simulink model "PMSM_drive_Simulink"  (R2024a)
settings: Solver=ode45  StartTime=0.0  StopTime=10.0  RelTol=1e-6  AbsTol=1e-8
values from neighbouring files (symbols this model uses):
  B = 0.08    [PMSM_drive_main_code.m]
  Ba = alfaw*J - B    (= 0.17)    [PMSM_drive_main_code.m]
  Beta0 = Beta_fixed*pi/180    (= 1.9753514301)    [PMSM_drive_main_code.m]
  Beta_step = 130*pi/180    (= 2.26892802759)    [PMSM_drive_main_code.m]
  Beta_time = 2.3    [PMSM_drive_main_code.m]
  Irated = 6.5*sqrt(2)    [PMSM_drive_main_code.m]
  isd0 = 0    [PMSM_drive_main_code.m]
  isq0 = 0    [PMSM_drive_main_code.m]
  J = 0.0125    [PMSM_drive_main_code.m]
  Kicd = alfac*(Rs+Rad)    (= 34500)    [PMSM_drive_main_code.m]
  Kicq = alfac*(Rs+Raq)    (= 85500)    [PMSM_drive_main_code.m]
  Kiw = alfaw*(B+Ba)    (= 5)    [PMSM_drive_main_code.m]
  Kpcd = alfac*Lsdhat    (= 34.5)    [PMSM_drive_main_code.m]
  Kpcq = alfac*Lsqhat    (= 85.5)    [PMSM_drive_main_code.m]
  Kpw = alfaw*J    (= 0.25)    [PMSM_drive_main_code.m]
  Lsd = Laa0+Lab0+3/2*Laa2    (= 0.0345)    [PMSM_drive_main_code.m]
  Lsq = Laa0+Lab0-3/2*Laa2    (= 0.0855)    [PMSM_drive_main_code.m]
  np = 2    [PMSM_drive_main_code.m]
  Psim = 0.822    [PMSM_drive_main_code.m]
  Rad = alfac*Lsdhat-Rs    (= 33.17)    [PMSM_drive_main_code.m]
  Raq = alfac*Lsqhat-Rs    (= 84.17)    [PMSM_drive_main_code.m]
  Rs = 1.33    [PMSM_drive_main_code.m]
  Te_ref = 16.6    [PMSM_drive_main_code.m]
  Te_ref2 = 4    [PMSM_drive_main_code.m]
  Te_ref_time = 0.1    [PMSM_drive_main_code.m]
  Te_ref_time2 = 2.7    [PMSM_drive_main_code.m]
  theta0 = 0    [PMSM_drive_main_code.m]
  TL_extra = 4    [PMSM_drive_main_code.m]
  TL_extra_time = 1.1    [PMSM_drive_main_code.m]
  Umax = 440*sqrt(2/3)    [PMSM_drive_main_code.m]
  usd0 = Rs*isd0-ws*Lsq*isq0    [PMSM_drive_main_code.m]
  usq0 = Rs*isq0+ws*Lsd*isd0+ws*Psim    [PMSM_drive_main_code.m]
  VconvLim = Umax    [PMSM_drive_main_code.m]
  wr0 = 0    [PMSM_drive_main_code.m]
  ws = 2*pi*fs    (= 314.159265359)    [PMSM_drive_main_code.m]
undefined symbols (not defined in the file or in its folder): j
settings Model: Creator=e6zebra  LastModifiedBy=munav
settings SolverCC: AutoScaleAbsTol=off  AlgebraicLoopSolver=TrustRegion
settings DataIOCC: SaveFormat=Array  SignalLoggingSaveFormat=ModelDataLogs  ReturnWorkspaceOutputs=off
settings OptimizationCC: BlockReduction=off  BooleanDataType=off  ExpressionDepthLimit=2147483647  InitFltsAndDblsToZero=on  LifeSpan=inf
settings DebuggingCC: SaveWithParameterizedLinksMsg=none  UnderspecifiedInitializationDetection=Classic  MergeDetectMultiDrivingBlocksExec=none  SignalResolutionControl=TryResolveAllWithWarning  MultiTaskDSMMsg=warning  MultiTaskCondExecSysMsg=none  FcnCallInpInsideContextMsg=warning  UnconnectedInputMsg=warning  UnconnectedOutputMsg=warning  UnconnectedLineMsg=warning  StateNameClashWarn=warning  SFUnexpectedBacktrackingDiag=warning  SFNoUnconditionalDefaultTransitionDiag=warning  SFExecutionAtInitializationDiag=none  ArithmeticOperatorsInVariantConditions=warning
settings HardwareCC: ProdBitPerPointer=32  ProdBitPerSizeT=32  ProdBitPerPtrDiffT=32  ProdLargestAtomicFloat=None  ProdIntDivRoundTo=Undefined  ProdEndianess=Unspecified  ProdWordSize=32  ProdHWDeviceType=32-bit Generic  TargetUnknown=on
settings ModelReferenceCC: EnableRefExpFcnMdlSchedulingChecks=on  PropagateSignalLabelsOutOfModel=off
settings SFSimCC: SimUseLocalCustomCode=off  CustomCodeUndefinedFunction=UseInterfaceOnly
settings RTWCC: TemplateMakefile=grt.tmf  RTWUseLocalCustomCode=off  GPUComputeCapability=3.5
settings CodeAppCC: StateflowObjectComments=on
settings GRTTargetCC: TargetFcnLib=ansi_tfl_tmw.mat  TargetLangStandard=C89/C90 (ANSI)  CombineOutputUpdateFcns=off  GRTInterface=on
settings ConfigComp: CovMetricSettings=dw  CovSaveCumulativeToWorkspaceVar=on  CovSaveSingleToWorkspaceVar=on  CovExternalEMLEnable=off

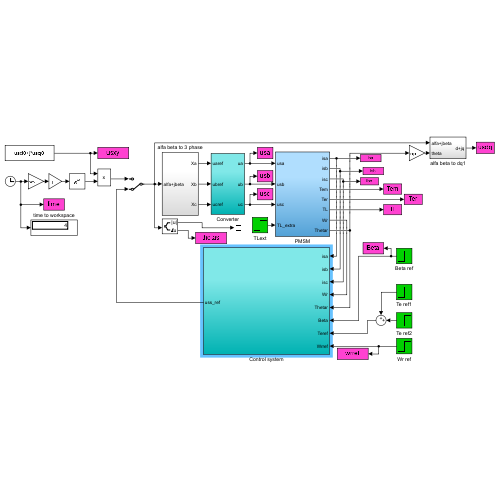
[thumbnail: Simulink's stored preview of the top-level diagram]
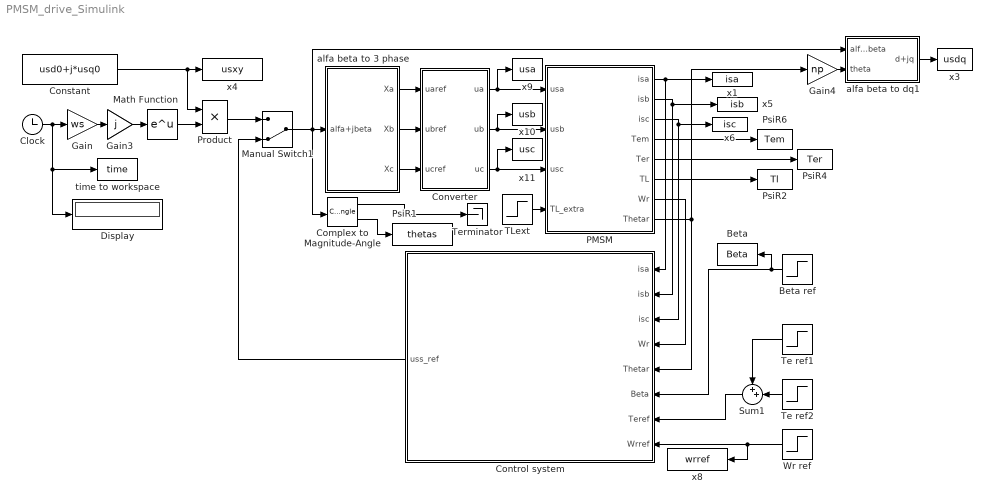
== system PMSM_drive_Simulink ==
  Beta : ToWorkspace  VariableName=Beta  SampleTime=-1
  Beta ref : Step  Time=Beta_time  Before=Beta0  After=Beta_step  SampleTime=0
  Clock : Clock
  Complex to Magnitude-Angle : ComplexToMagnitudeAngle
  Constant : Constant  Value=usd0+j*usq0
  Control system : Subsystem
  Converter : Subsystem
  Display : Display
  Gain : Gain  Gain=ws
  Gain3 : Gain  Gain=j  SaturateOnIntegerOverflow=on  OutDataTypeStr=Inherit: Same as input  ParamDataTypeStr=Inherit: Same as input
  Gain4 : Gain  Gain=np
  Manual Switch1 : ManualSwitch  CurrentSetting=0
  Math Function : Math  SignedPower=on
  PMSM : Subsystem
  Product : Product  SaturateOnIntegerOverflow=on  OutDataTypeStr=Inherit: Same as first input
  PsiR1 : ToWorkspace  VariableName=thetas  SampleTime=-1
  PsiR2 : ToWorkspace  VariableName=Tl  SampleTime=-1
  PsiR4 : ToWorkspace  VariableName=Ter  SampleTime=-1
  PsiR6 : ToWorkspace  VariableName=Tem  SampleTime=-1
  Sum1 : Sum  Inputs=++|  SaturateOnIntegerOverflow=on
  TLext : Step  Time=TL_extra_time  After=TL_extra  SampleTime=0
  Te ref1 : Step  Time=Te_ref_time  After=Te_ref  SampleTime=0
  Te ref2 : Step  Time=Te_ref_time2  After=Te_ref2  SampleTime=0
  Terminator : Terminator
  Wr ref : Step  After=1435*pi/30  SampleTime=0
  alfa beta to 3 phase : Subsystem
  alfa beta to dq1 : Subsystem
  time to workspace : ToWorkspace  VariableName=time  SampleTime=-1
  x1 : ToWorkspace  VariableName=isa  SampleTime=-1
  x10 : ToWorkspace  VariableName=usb  SampleTime=-1
  x11 : ToWorkspace  VariableName=usc  SampleTime=-1
  x3 : ToWorkspace  VariableName=usdq  SampleTime=-1
  x4 : ToWorkspace  VariableName=usxy  SampleTime=-1
  x5 : ToWorkspace  VariableName=isb  SampleTime=-1
  x6 : ToWorkspace  VariableName=isc  SampleTime=-1
  x8 : ToWorkspace  VariableName=wrref  SampleTime=-1
  x9 : ToWorkspace  VariableName=usa  SampleTime=-1
  wires:
  Clock/1 -> Gain/1, time to workspace/1, Display/1
  TLext/1 -> PMSM/4(TL_extra)
  Beta ref/1 -> Control system/6(Beta), Beta/1
  Wr ref/1 -> x8/1, Control system/8(Wrref)
  Gain/1 -> Gain3/1
  Constant/1 -> x4/1, Product/1
  PMSM/8(Thetar) -> Control system/5(Thetar), Gain4/1
  PMSM/6(TL) -> PsiR2/1
  PMSM/5(Ter) -> PsiR4/1
  alfa beta to dq1/1(d+jq) -> x3/1
  Converter/1(ua) -> PMSM/1(usa), x9/1
  Converter/2(ub) -> PMSM/2(usb), x10/1
  Converter/3(uc) -> PMSM/3(usc), x11/1
  alfa beta to 3 phase/1(Xa) -> Converter/1(uaref)
  alfa beta to 3 phase/2(Xb) -> Converter/2(ubref)
  alfa beta to 3 phase/3(Xc) -> Converter/3(ucref)
  Gain3/1 -> Math Function/1
  Math Function/1 -> Product/2
  Complex to Magnitude-Angle/2 -> PsiR1/1
  Complex to Magnitude-Angle/1 -> Terminator/1
  Te ref1/1 -> Sum1/1
  Te ref2/1 -> Sum1/2
  Manual Switch1/1 -> alfa beta to 3 phase/1(alfa+jbeta), alfa beta to dq1/1(alfa+jbeta), Complex to Magnitude-Angle/1
  PMSM/4(Tem) -> PsiR6/1
  Product/1 -> Manual Switch1/1
  Gain4/1 -> alfa beta to dq1/2(theta)
  PMSM/2(isb) -> Control system/2(isb), x5/1
  PMSM/3(isc) -> Control system/3(isc), x6/1
  PMSM/7(Wr) -> Control system/4(Wr)
  Sum1/1 -> Control system/7(Teref)
  Control system/1(uss_ref) -> Manual Switch1/2
  PMSM/1(isa) -> Control system/1(isa), x1/1

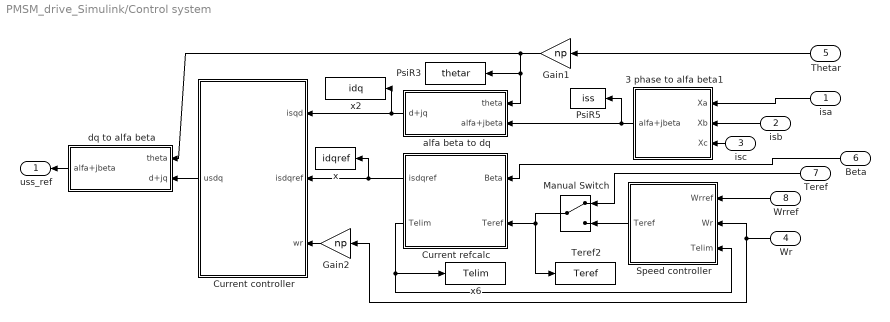
== system PMSM_drive_Simulink/Control system ==
  isa : Inport
  isb : Inport  Port=2
  isc : Inport  Port=3
  Wr : Inport  Port=4
  Thetar : Inport  Port=5
  Beta : Inport  Port=6
  Teref : Inport  Port=7
  Wrref : Inport  Port=8
  3 phase to alfa beta1 : Subsystem
  Current controller : Subsystem
  Current refcalc : Subsystem
  Gain1 : Gain  Gain=np
  Gain2 : Gain  Gain=np
  Manual Switch : ManualSwitch
  PsiR3 : ToWorkspace  VariableName=thetar  SampleTime=-1
  PsiR5 : ToWorkspace  VariableName=iss  SampleTime=-1
  Speed controller : Subsystem
  Teref2 : ToWorkspace  VariableName=Teref  SampleTime=-1
  alfa beta to dq : Subsystem
  dq to alfa beta : Subsystem
  x : ToWorkspace  VariableName=idqref  SampleTime=-1
  x2 : ToWorkspace  VariableName=idq  SampleTime=-1
  x6 : ToWorkspace  VariableName=Telim  SampleTime=-1
  uss_ref : Outport  VectorParamsAs1DForOutWhenUnconnected=off
  wires:
  Wr/1 -> Gain2/1, Speed controller/2(Wr)
  alfa beta to dq/1(d+jq) -> x2/1, Current controller/1(isqd)
  Current refcalc/1(isdqref) -> x/1, Current controller/2(isdqref)
  Current refcalc/2(Telim) -> Speed controller/3(Telim), x6/1
  Gain1/1 -> PsiR3/1, alfa beta to dq/1(theta), dq to alfa beta/1(theta)
  Gain2/1 -> Current controller/3(wr)
  isc/1 -> 3 phase to alfa beta1/3(Xc)
  isb/1 -> 3 phase to alfa beta1/2(Xb)
  isa/1 -> 3 phase to alfa beta1/1(Xa)
  3 phase to alfa beta1/1(alfa+jbeta) -> PsiR5/1, alfa beta to dq/2(alfa+jbeta)
  Current controller/1(usdq) -> dq to alfa beta/2(d+jq)
  Manual Switch/1 -> Current refcalc/2(Teref), Teref2/1
  dq to alfa beta/1(alfa+jbeta) -> uss_ref/1
  Thetar/1 -> Gain1/1
  Beta/1 -> Current refcalc/1(Beta)
  Wrref/1 -> Speed controller/1(Wrref)
  Teref/1 -> Manual Switch/1
  Speed controller/1(Teref) -> Manual Switch/2

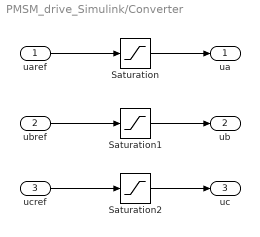
== system PMSM_drive_Simulink/Converter ==
  uaref : Inport
  ubref : Inport  Port=2
  ucref : Inport  Port=3
  Saturation : Saturate  UpperLimit=VconvLim  LowerLimit=-VconvLim
  Saturation1 : Saturate  UpperLimit=VconvLim  LowerLimit=-VconvLim
  Saturation2 : Saturate  UpperLimit=VconvLim  LowerLimit=-VconvLim
  ua : Outport  VectorParamsAs1DForOutWhenUnconnected=off
  ub : Outport  Port=2  VectorParamsAs1DForOutWhenUnconnected=off
  uc : Outport  Port=3  VectorParamsAs1DForOutWhenUnconnected=off
  wires:
  Saturation2/1 -> uc/1
  Saturation1/1 -> ub/1
  Saturation/1 -> ua/1
  uaref/1 -> Saturation/1
  ubref/1 -> Saturation1/1
  ucref/1 -> Saturation2/1

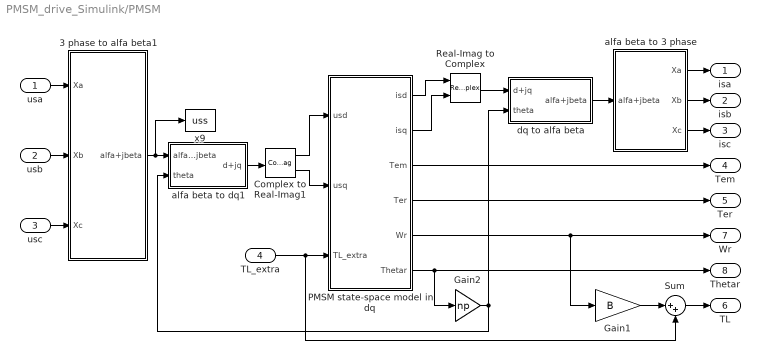
== system PMSM_drive_Simulink/PMSM ==
  usa : Inport
  usb : Inport  Port=2
  usc : Inport  Port=3
  TL_extra : Inport  Port=4
  3 phase to alfa beta1 : Subsystem
  Complex to Real-Imag1 : ComplexToRealImag
  Gain1 : Gain  Gain=B
  Gain2 : Gain  Gain=np
  PMSM state-space model in dq : Subsystem
  Real-Imag to Complex : RealImagToComplex
  Sum : Sum  Inputs=|++  SaturateOnIntegerOverflow=on
  alfa beta to 3 phase : Subsystem
  alfa beta to dq1 : Subsystem
  dq to alfa beta : Subsystem
  x9 : ToWorkspace  VariableName=uss  SampleTime=-1
  isa : Outport  VectorParamsAs1DForOutWhenUnconnected=off
  isb : Outport  Port=2  VectorParamsAs1DForOutWhenUnconnected=off
  isc : Outport  Port=3  VectorParamsAs1DForOutWhenUnconnected=off
  Tem : Outport  Port=4  VectorParamsAs1DForOutWhenUnconnected=off
  Ter : Outport  Port=5  VectorParamsAs1DForOutWhenUnconnected=off
  TL : Outport  Port=6  VectorParamsAs1DForOutWhenUnconnected=off
  Wr : Outport  Port=7  VectorParamsAs1DForOutWhenUnconnected=off
  Thetar : Outport  Port=8  VectorParamsAs1DForOutWhenUnconnected=off
  wires:
  TL_extra/1 -> Sum/2, PMSM state-space model in dq/3(TL_extra)
  Gain1/1 -> Sum/1
  Sum/1 -> TL/1
  usc/1 -> 3 phase to alfa beta1/3(Xc)
  usb/1 -> 3 phase to alfa beta1/2(Xb)
  usa/1 -> 3 phase to alfa beta1/1(Xa)
  alfa beta to 3 phase/1(Xa) -> isa/1
  alfa beta to 3 phase/3(Xc) -> isc/1
  alfa beta to 3 phase/2(Xb) -> isb/1
  Real-Imag to Complex/1 -> dq to alfa beta/1(d+jq)
  dq to alfa beta/1(alfa+jbeta) -> alfa beta to 3 phase/1(alfa+jbeta)
  alfa beta to dq1/1(d+jq) -> Complex to Real-Imag1/1
  PMSM state-space model in dq/5(Wr) -> Gain1/1, Wr/1
  PMSM state-space model in dq/6(Thetar) -> Gain2/1, Thetar/1
  Complex to Real-Imag1/1 -> PMSM state-space model in dq/1(usd)
  Complex to Real-Imag1/2 -> PMSM state-space model in dq/2(usq)
  PMSM state-space model in dq/1(isd) -> Real-Imag to Complex/1
  PMSM state-space model in dq/2(isq) -> Real-Imag to Complex/2
  PMSM state-space model in dq/3(Tem) -> Tem/1
  PMSM state-space model in dq/4(Ter) -> Ter/1
  Gain2/1 -> alfa beta to dq1/2(theta), dq to alfa beta/2(theta)
  3 phase to alfa beta1/1(alfa+jbeta) -> x9/1, alfa beta to dq1/1(alfa+jbeta)

== system PMSM_drive_Simulink/alfa beta to 3 phase ==
  alfa+jbeta : Inport
  Add1 : Sum  Inputs=-+
  Add2 : Sum  Inputs=--
  Complex to Real-Imag : ComplexToRealImag
  Gain1 : Gain  Gain=sqrt(3)/2
  Gain2 : Gain  Gain=1/2
  Xa : Outport  VectorParamsAs1DForOutWhenUnconnected=off
  Xb : Outport  Port=2  VectorParamsAs1DForOutWhenUnconnected=off
  Xc : Outport  Port=3  VectorParamsAs1DForOutWhenUnconnected=off
  wires:
  alfa+jbeta/1 -> Complex to Real-Imag/1
  Complex to Real-Imag/1 -> Xa/1, Gain2/1
  Add2/1 -> Xc/1
  Add1/1 -> Xb/1
  Complex to Real-Imag/2 -> Gain1/1
  Gain1/1 -> Add1/2, Add2/2
  Gain2/1 -> Add1/1, Add2/1

== system PMSM_drive_Simulink/alfa beta to dq1 ==
  alfa+jbeta : Inport
  theta : Inport  Port=2
  Gain : Gain  Gain=-j  SaturateOnIntegerOverflow=on  OutDataTypeStr=Inherit: Same as input  ParamDataTypeStr=Inherit: Same as input
  Math Function : Math  SignedPower=on
  Product : Product  SaturateOnIntegerOverflow=on  OutDataTypeStr=Inherit: Same as first input
  d+jq : Outport  VectorParamsAs1DForOutWhenUnconnected=off
  wires:
  theta/1 -> Gain/1
  Gain/1 -> Math Function/1
  Math Function/1 -> Product/2
  alfa+jbeta/1 -> Product/1
  Product/1 -> d+jq/1

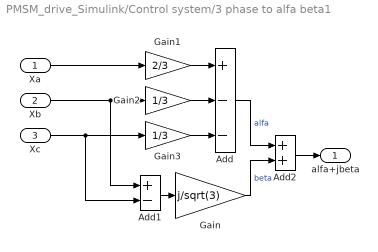
== system PMSM_drive_Simulink/Control system/3 phase to alfa beta1 ==
  Xa : Inport
  Xb : Inport  Port=2
  Xc : Inport  Port=3
  Add : Sum  Inputs=+--
  Add1 : Sum  Inputs=+-
  Add2 : Sum
  Gain : Gain  Gain=j/sqrt(3)
  Gain1 : Gain  Gain=2/3
  Gain2 : Gain  Gain=1/3
  Gain3 : Gain  Gain=1/3
  alfa+jbeta : Outport  VectorParamsAs1DForOutWhenUnconnected=off
  wires:
  Add1/1 -> Gain/1
  Add2/1 -> alfa+jbeta/1
  Gain/1 -> Add2/2  "beta"
  Add/1 -> Add2/1  "alfa"
  Gain3/1 -> Add/3
  Gain2/1 -> Add/2
  Gain1/1 -> Add/1
  Xa/1 -> Gain1/1
  Xb/1 -> Gain2/1, Add1/1
  Xc/1 -> Gain3/1, Add1/2

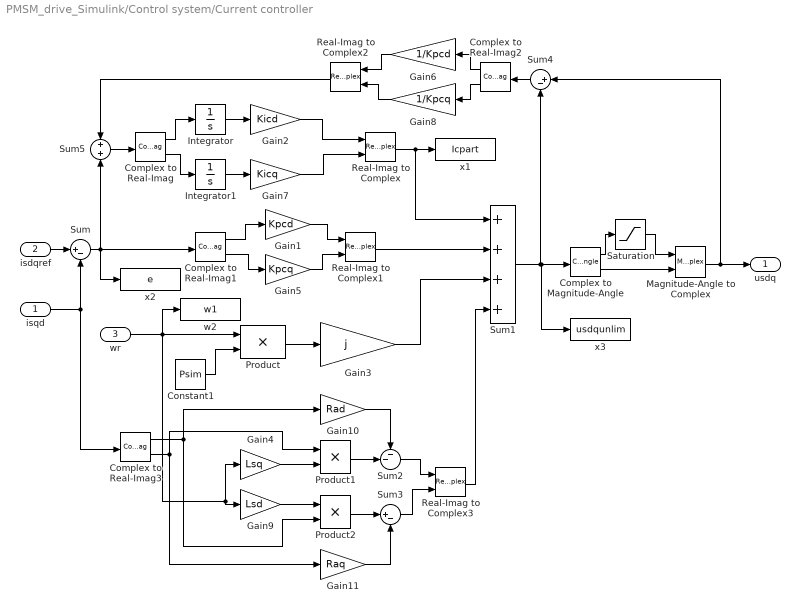
== system PMSM_drive_Simulink/Control system/Current controller ==
  isqd : Inport
  isdqref : Inport  Port=2
  wr : Inport  Port=3
  Complex to Magnitude-Angle : ComplexToMagnitudeAngle
  Complex to Real-Imag{,1..3} (4 alike) : ComplexToRealImag
  Constant1 : Constant  Value=Psim
  Gain1 : Gain  Gain=Kpcd  SaturateOnIntegerOverflow=on  OutDataTypeStr=Inherit: Same as input  ParamDataTypeStr=Inherit: Same as input
  Gain10 : Gain  Gain=Rad  SaturateOnIntegerOverflow=on  OutDataTypeStr=Inherit: Same as input  ParamDataTypeStr=Inherit: Same as input
  Gain11 : Gain  Gain=Raq  SaturateOnIntegerOverflow=on  OutDataTypeStr=Inherit: Same as input  ParamDataTypeStr=Inherit: Same as input
  Gain2 : Gain  Gain=Kicd  SaturateOnIntegerOverflow=on  OutDataTypeStr=Inherit: Same as input  ParamDataTypeStr=Inherit: Same as input
  Gain3 : Gain  Gain=j  SaturateOnIntegerOverflow=on  OutDataTypeStr=Inherit: Same as input  ParamDataTypeStr=Inherit: Same as input
  Gain4 : Gain  Gain=Lsq  SaturateOnIntegerOverflow=on  OutDataTypeStr=Inherit: Same as input  ParamDataTypeStr=Inherit: Same as input
  Gain5 : Gain  Gain=Kpcq  SaturateOnIntegerOverflow=on  OutDataTypeStr=Inherit: Same as input  ParamDataTypeStr=Inherit: Same as input
  Gain6 : Gain  Gain=1/Kpcd  SaturateOnIntegerOverflow=on  OutDataTypeStr=Inherit: Same as input  ParamDataTypeStr=Inherit: Same as input
  Gain7 : Gain  Gain=Kicq  SaturateOnIntegerOverflow=on  OutDataTypeStr=Inherit: Same as input  ParamDataTypeStr=Inherit: Same as input
  Gain8 : Gain  Gain=1/Kpcq  SaturateOnIntegerOverflow=on  OutDataTypeStr=Inherit: Same as input  ParamDataTypeStr=Inherit: Same as input
  Gain9 : Gain  Gain=Lsd  SaturateOnIntegerOverflow=on  OutDataTypeStr=Inherit: Same as input  ParamDataTypeStr=Inherit: Same as input
  Integrator : Integrator
  Integrator1 : Integrator
  Magnitude-Angle to Complex : MagnitudeAngleToComplex
  Product : Product  SaturateOnIntegerOverflow=on  OutDataTypeStr=Inherit: Same as first input
  Product1 : Product  SaturateOnIntegerOverflow=on  OutDataTypeStr=Inherit: Same as first input
  Product2 : Product  SaturateOnIntegerOverflow=on  OutDataTypeStr=Inherit: Same as first input
  Real-Imag to Complex{,1..3} (4 alike) : RealImagToComplex
  Saturation : Saturate  UpperLimit=Umax  LowerLimit=0
  Sum : Sum  Inputs=|+-  SaturateOnIntegerOverflow=on
  Sum1 : Sum  Inputs=++++  SaturateOnIntegerOverflow=on
  Sum2 : Sum  Inputs=--|  SaturateOnIntegerOverflow=on
  Sum3 : Sum  Inputs=|+-  SaturateOnIntegerOverflow=on
  Sum4 : Sum  Inputs=|+-  SaturateOnIntegerOverflow=on
  Sum5 : Sum  SaturateOnIntegerOverflow=on
  w2 : ToWorkspace  VariableName=w1  SampleTime=-1
  x1 : ToWorkspace  VariableName=Icpart  SampleTime=-1
  x2 : ToWorkspace  VariableName=e  SampleTime=-1
  x3 : ToWorkspace  VariableName=usdqunlim  SampleTime=-1
  usdq : Outport  VectorParamsAs1DForOutWhenUnconnected=off
  wires:
  isdqref/1 -> Sum/1
  isqd/1 -> Sum/2, Complex to Real-Imag3/1
  Sum/1 -> x2/1, Complex to Real-Imag1/1, Sum5/2
  Sum1/1 -> Complex to Magnitude-Angle/1, x3/1, Sum4/2
  Complex to Magnitude-Angle/1 -> Saturation/1
  Saturation/1 -> Magnitude-Angle to Complex/1
  Complex to Magnitude-Angle/2 -> Magnitude-Angle to Complex/2
  Magnitude-Angle to Complex/1 -> usdq/1, Sum4/1
  Complex to Real-Imag/2 -> Integrator1/1
  Complex to Real-Imag/1 -> Integrator/1
  Integrator/1 -> Gain2/1
  Integrator1/1 -> Gain7/1
  Real-Imag to Complex/1 -> Sum1/1, x1/1
  Product/1 -> Gain3/1
  Constant1/1 -> Product/2
  Gain4/1 -> Product1/2
  Gain3/1 -> Sum1/3
  Sum4/1 -> Complex to Real-Imag2/1
  Sum5/1 -> Complex to Real-Imag/1
  Real-Imag to Complex2/1 -> Sum5/1
  Complex to Real-Imag1/1 -> Gain1/1
  Real-Imag to Complex1/1 -> Sum1/2
  Gain1/1 -> Real-Imag to Complex1/1
  Complex to Real-Imag1/2 -> Gain5/1
  Gain5/1 -> Real-Imag to Complex1/2
  Gain2/1 -> Real-Imag to Complex/1
  Gain7/1 -> Real-Imag to Complex/2
  Complex to Real-Imag2/1 -> Gain6/1
  Gain6/1 -> Real-Imag to Complex2/1
  Complex to Real-Imag2/2 -> Gain8/1
  Gain8/1 -> Real-Imag to Complex2/2
  wr/1 -> w2/1, Gain4/1, Gain9/1, Product/1
  Real-Imag to Complex3/1 -> Sum1/4
  Complex to Real-Imag3/2 -> Product1/1, Gain11/1
  Sum2/1 -> Real-Imag to Complex3/1
  Gain9/1 -> Product2/1
  Complex to Real-Imag3/1 -> Product2/2, Gain10/1
  Product1/1 -> Sum2/2
  Gain10/1 -> Sum2/1
  Product2/1 -> Sum3/1
  Sum3/1 -> Real-Imag to Complex3/2
  Gain11/1 -> Sum3/2

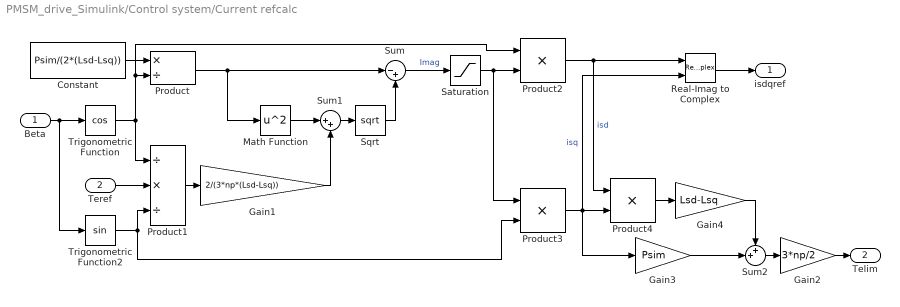
== system PMSM_drive_Simulink/Control system/Current refcalc ==
  Beta : Inport
  Teref : Inport  Port=2
  Constant : Constant  Value=Psim/(2*(Lsd-Lsq))
  Gain1 : Gain  Gain=2/(3*np*(Lsd-Lsq))  SaturateOnIntegerOverflow=on  OutDataTypeStr=Inherit: Same as input  ParamDataTypeStr=Inherit: Same as input
  Gain2 : Gain  Gain=3*np/2  SaturateOnIntegerOverflow=on  OutDataTypeStr=Inherit: Same as input  ParamDataTypeStr=Inherit: Same as input
  Gain3 : Gain  Gain=Psim  SaturateOnIntegerOverflow=on  OutDataTypeStr=Inherit: Same as input  ParamDataTypeStr=Inherit: Same as input
  Gain4 : Gain  Gain=Lsd-Lsq  SaturateOnIntegerOverflow=on  OutDataTypeStr=Inherit: Same as input  ParamDataTypeStr=Inherit: Same as input
  Math Function : Math  Operator=square  SignedPower=on
  Product : Product  Inputs=*/  SaturateOnIntegerOverflow=on  OutDataTypeStr=Inherit: Same as first input
  Product1 : Product  Inputs=/*/  SaturateOnIntegerOverflow=on  OutDataTypeStr=Inherit: Same as first input
  Product2 : Product  Inputs=**  SaturateOnIntegerOverflow=on  OutDataTypeStr=Inherit: Same as first input
  Product3 : Product  Inputs=**  SaturateOnIntegerOverflow=on  OutDataTypeStr=Inherit: Same as first input
  Product4 : Product  Inputs=**  SaturateOnIntegerOverflow=on  OutDataTypeStr=Inherit: Same as first input
  Real-Imag to Complex : RealImagToComplex
  Saturation : Saturate  UpperLimit=Irated  LowerLimit=0
  Sqrt : Sqrt
  Sum : Sum  Inputs=|-+
  Sum1 : Sum  Inputs=|++
  Sum2 : Sum  Inputs=++|
  Trigonometric Function : Trigonometry  Operator=cos
  Trigonometric Function2 : Trigonometry
  isdqref : Outport  VectorParamsAs1DForOutWhenUnconnected=off
  Telim : Outport  Port=2  VectorParamsAs1DForOutWhenUnconnected=off
  wires:
  Constant/1 -> Product/1
  Trigonometric Function/1 -> Product2/1, Product/2, Product1/1
  Beta/1 -> Trigonometric Function/1, Trigonometric Function2/1
  Product/1 -> Math Function/1, Sum/1
  Sqrt/1 -> Sum/2
  Sum1/1 -> Sqrt/1
  Math Function/1 -> Sum1/1
  Trigonometric Function2/1 -> Product1/3, Product3/2
  Teref/1 -> Product1/2
  Product1/1 -> Gain1/1
  Gain1/1 -> Sum1/2
  Sum/1 -> Saturation/1  "Imag"
  Product2/1 -> Product4/1, Real-Imag to Complex/1  "isd"
  Product3/1 -> Product4/2, Real-Imag to Complex/2, Gain3/1  "isq"
  Real-Imag to Complex/1 -> isdqref/1
  Saturation/1 -> Product2/2, Product3/1
  Gain2/1 -> Telim/1
  Sum2/1 -> Gain2/1
  Product4/1 -> Gain4/1
  Gain3/1 -> Sum2/2
  Gain4/1 -> Sum2/1

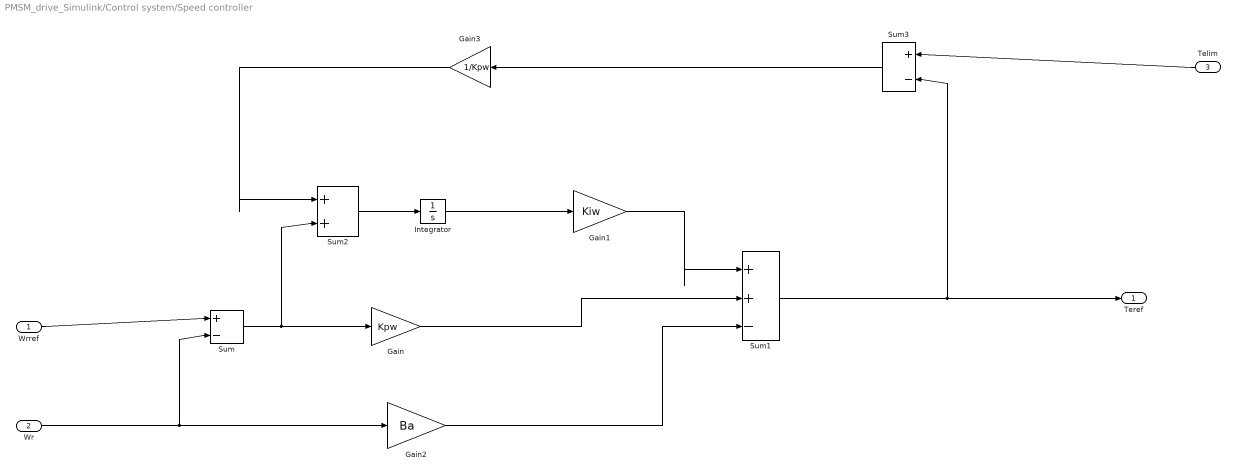
== system PMSM_drive_Simulink/Control system/Speed controller ==
  Wrref : Inport
  Wr : Inport  Port=2
  Telim : Inport  Port=3
  Gain : Gain  Gain=Kpw
  Gain1 : Gain  Gain=Kiw
  Gain2 : Gain  Gain=Ba
  Gain3 : Gain  Gain=1/Kpw
  Integrator : Integrator
  Sum : Sum  Inputs=|+-
  Sum1 : Sum  Inputs=|++-
  Sum2 : Sum  Inputs=|++
  Sum3 : Sum  Inputs=|+-
  Teref : Outport  VectorParamsAs1DForOutWhenUnconnected=off
  wires:
  Wrref/1 -> Sum/1
  Telim/1 -> Sum3/1
  Wr/1 -> Sum/2, Gain2/1
  Sum1/1 -> Teref/1, Sum3/2
  Sum/1 -> Gain/1, Sum2/2
  Gain3/1 -> Sum2/1
  Gain/1 -> Sum1/2
  Gain2/1 -> Sum1/3
  Sum3/1 -> Gain3/1
  Sum2/1 -> Integrator/1
  Integrator/1 -> Gain1/1
  Gain1/1 -> Sum1/1

== system PMSM_drive_Simulink/Control system/alfa beta to dq ==
  theta : Inport
  alfa+jbeta : Inport  Port=2
  Gain : Gain  Gain=-j  SaturateOnIntegerOverflow=on  OutDataTypeStr=Inherit: Same as input  ParamDataTypeStr=Inherit: Same as input
  Math Function : Math  SignedPower=on
  Product : Product  SaturateOnIntegerOverflow=on  OutDataTypeStr=Inherit: Same as first input
  d+jq : Outport  VectorParamsAs1DForOutWhenUnconnected=off
  wires:
  theta/1 -> Gain/1
  Gain/1 -> Math Function/1
  Math Function/1 -> Product/2
  alfa+jbeta/1 -> Product/1
  Product/1 -> d+jq/1

== system PMSM_drive_Simulink/Control system/dq to alfa beta ==
  theta : Inport
  d+jq : Inport  Port=2
  Gain : Gain  Gain=j  SaturateOnIntegerOverflow=on  OutDataTypeStr=Inherit: Same as input  ParamDataTypeStr=Inherit: Same as input
  Math Function : Math  SignedPower=on
  Product : Product  SaturateOnIntegerOverflow=on  OutDataTypeStr=Inherit: Same as first input
  alfa+jbeta : Outport  VectorParamsAs1DForOutWhenUnconnected=off
  wires:
  theta/1 -> Gain/1
  Gain/1 -> Math Function/1
  Math Function/1 -> Product/2
  d+jq/1 -> Product/1
  Product/1 -> alfa+jbeta/1

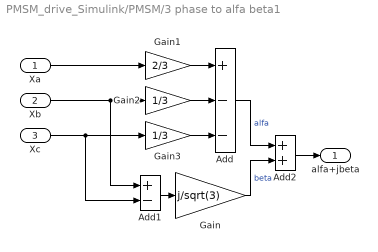
== system PMSM_drive_Simulink/PMSM/3 phase to alfa beta1 ==
  Xa : Inport
  Xb : Inport  Port=2
  Xc : Inport  Port=3
  Add : Sum  Inputs=+--
  Add1 : Sum  Inputs=+-
  Add2 : Sum
  Gain : Gain  Gain=j/sqrt(3)
  Gain1 : Gain  Gain=2/3
  Gain2 : Gain  Gain=1/3
  Gain3 : Gain  Gain=1/3
  alfa+jbeta : Outport  VectorParamsAs1DForOutWhenUnconnected=off
  wires:
  Add1/1 -> Gain/1
  Add2/1 -> alfa+jbeta/1
  Gain/1 -> Add2/2  "beta"
  Add/1 -> Add2/1  "alfa"
  Gain3/1 -> Add/3
  Gain2/1 -> Add/2
  Gain1/1 -> Add/1
  Xa/1 -> Gain1/1
  Xb/1 -> Gain2/1, Add1/1
  Xc/1 -> Gain3/1, Add1/2

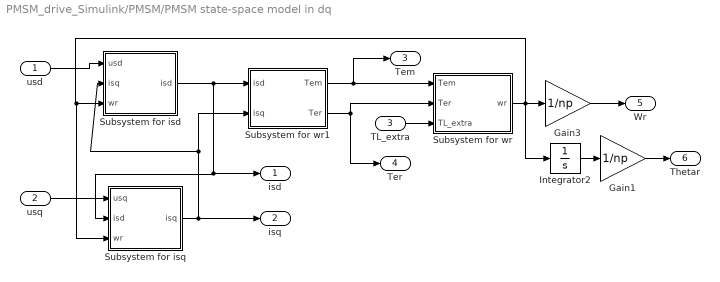
== system PMSM_drive_Simulink/PMSM/PMSM state-space model in dq ==
  usd : Inport
  usq : Inport  Port=2
  TL_extra : Inport  Port=3
  Gain1 : Gain  Gain=1/np
  Gain3 : Gain  Gain=1/np
  Integrator2 : Integrator  InitialCondition=theta0
  Subsystem for isd : Subsystem
  Subsystem for isq : Subsystem
  Subsystem for wr : Subsystem
  Subsystem for wr1 : Subsystem
  isd : Outport  VectorParamsAs1DForOutWhenUnconnected=off
  isq : Outport  Port=2  VectorParamsAs1DForOutWhenUnconnected=off
  Tem : Outport  Port=3  VectorParamsAs1DForOutWhenUnconnected=off
  Ter : Outport  Port=4  VectorParamsAs1DForOutWhenUnconnected=off
  Wr : Outport  Port=5  VectorParamsAs1DForOutWhenUnconnected=off
  Thetar : Outport  Port=6  VectorParamsAs1DForOutWhenUnconnected=off
  wires:
  Subsystem for isq/1(isq) -> isq/1, Subsystem for wr1/2(isq), Subsystem for isd/2(isq)
  usd/1 -> Subsystem for isd/1(usd)
  Subsystem for isd/1(isd) -> isd/1, Subsystem for isq/2(isd), Subsystem for wr1/1(isd)
  usq/1 -> Subsystem for isq/1(usq)
  Gain3/1 -> Wr/1
  Integrator2/1 -> Gain1/1
  TL_extra/1 -> Subsystem for wr/3(TL_extra)
  Subsystem for wr1/2(Ter) -> Ter/1, Subsystem for wr/2(Ter)
  Subsystem for wr1/1(Tem) -> Tem/1, Subsystem for wr/1(Tem)
  Subsystem for wr/1(wr) -> Integrator2/1, Gain3/1, Subsystem for isq/3(wr), Subsystem for isd/3(wr)
  Gain1/1 -> Thetar/1

== system PMSM_drive_Simulink/PMSM/alfa beta to 3 phase ==
  alfa+jbeta : Inport
  Add1 : Sum  Inputs=-+
  Add2 : Sum  Inputs=--
  Complex to Real-Imag : ComplexToRealImag
  Gain1 : Gain  Gain=sqrt(3)/2
  Gain2 : Gain  Gain=1/2
  Xa : Outport  VectorParamsAs1DForOutWhenUnconnected=off
  Xb : Outport  Port=2  VectorParamsAs1DForOutWhenUnconnected=off
  Xc : Outport  Port=3  VectorParamsAs1DForOutWhenUnconnected=off
  wires:
  alfa+jbeta/1 -> Complex to Real-Imag/1
  Complex to Real-Imag/1 -> Xa/1, Gain2/1
  Add2/1 -> Xc/1
  Add1/1 -> Xb/1
  Complex to Real-Imag/2 -> Gain1/1
  Gain1/1 -> Add1/2, Add2/2
  Gain2/1 -> Add1/1, Add2/1

== system PMSM_drive_Simulink/PMSM/alfa beta to dq1 ==
  alfa+jbeta : Inport
  theta : Inport  Port=2
  Gain : Gain  Gain=-j  SaturateOnIntegerOverflow=on  OutDataTypeStr=Inherit: Same as input  ParamDataTypeStr=Inherit: Same as input
  Math Function : Math  SignedPower=on
  Product : Product  SaturateOnIntegerOverflow=on  OutDataTypeStr=Inherit: Same as first input
  d+jq : Outport  VectorParamsAs1DForOutWhenUnconnected=off
  wires:
  theta/1 -> Gain/1
  Gain/1 -> Math Function/1
  Math Function/1 -> Product/2
  alfa+jbeta/1 -> Product/1
  Product/1 -> d+jq/1

== system PMSM_drive_Simulink/PMSM/dq to alfa beta ==
  d+jq : Inport
  theta : Inport  Port=2
  Gain : Gain  Gain=j  SaturateOnIntegerOverflow=on  OutDataTypeStr=Inherit: Same as input  ParamDataTypeStr=Inherit: Same as input
  Math Function : Math  SignedPower=on
  Product : Product  SaturateOnIntegerOverflow=on  OutDataTypeStr=Inherit: Same as first input
  alfa+jbeta : Outport  VectorParamsAs1DForOutWhenUnconnected=off
  wires:
  theta/1 -> Gain/1
  Gain/1 -> Math Function/1
  Math Function/1 -> Product/2
  d+jq/1 -> Product/1
  Product/1 -> alfa+jbeta/1

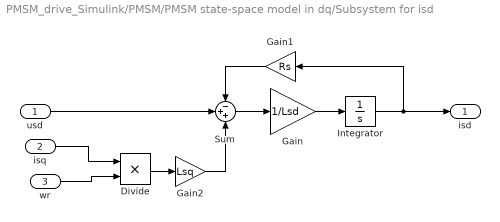
== system PMSM_drive_Simulink/PMSM/PMSM state-space model in dq/Subsystem for isd ==
  usd : Inport
  isq : Inport  Port=2
  wr : Inport  Port=3
  Divide : Product  Inputs=**
  Gain : Gain  Gain=1/Lsd
  Gain1 : Gain  Gain=Rs
  Gain2 : Gain  Gain=Lsq
  Integrator : Integrator  InitialCondition=isd0
  Sum : Sum  Inputs=-++
  isd : Outport  VectorParamsAs1DForOutWhenUnconnected=off
  wires:
  wr/1 -> Divide/2
  Divide/1 -> Gain2/1
  Gain2/1 -> Sum/3
  Gain/1 -> Integrator/1
  Integrator/1 -> isd/1, Gain1/1
  usd/1 -> Sum/2
  Gain1/1 -> Sum/1
  Sum/1 -> Gain/1
  isq/1 -> Divide/1

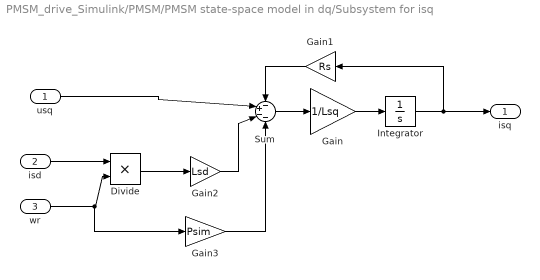
== system PMSM_drive_Simulink/PMSM/PMSM state-space model in dq/Subsystem for isq ==
  usq : Inport
  isd : Inport  Port=2
  wr : Inport  Port=3
  Divide : Product  Inputs=**
  Gain : Gain  Gain=1/Lsq
  Gain1 : Gain  Gain=Rs
  Gain2 : Gain  Gain=Lsd
  Gain3 : Gain  Gain=Psim
  Integrator : Integrator  InitialCondition=isq0
  Sum : Sum  Inputs=-+--
  isq : Outport  VectorParamsAs1DForOutWhenUnconnected=off
  wires:
  wr/1 -> Gain3/1, Divide/2
  Divide/1 -> Gain2/1
  Gain2/1 -> Sum/3
  Gain/1 -> Integrator/1
  Integrator/1 -> isq/1, Gain1/1
  usq/1 -> Sum/2
  Gain1/1 -> Sum/1
  Sum/1 -> Gain/1
  isd/1 -> Divide/1
  Gain3/1 -> Sum/4

== system PMSM_drive_Simulink/PMSM/PMSM state-space model in dq/Subsystem for wr ==
  Tem : Inport
  Ter : Inport  Port=2
  TL_extra : Inport  Port=3
  Gain : Gain  Gain=np/J
  Gain1 : Gain  Gain=B/np
  Integrator2 : Integrator  InitialCondition=wr0
  Sum : Sum  Inputs=++--
  wr : Outport  VectorParamsAs1DForOutWhenUnconnected=off
  wires:
  Integrator2/1 -> Gain1/1, wr/1
  Tem/1 -> Sum/1
  Ter/1 -> Sum/2
  TL_extra/1 -> Sum/3
  Sum/1 -> Gain/1
  Gain/1 -> Integrator2/1
  Gain1/1 -> Sum/4

== system PMSM_drive_Simulink/PMSM/PMSM state-space model in dq/Subsystem for wr1 ==
  isd : Inport
  isq : Inport  Port=2
  Divide : Product  Inputs=**
  Gain : Gain  Gain=3*np/2*Psim
  Gain1 : Gain  Gain=3*np/2*(Lsd-Lsq)
  Tem : Outport  VectorParamsAs1DForOutWhenUnconnected=off
  Ter : Outport  Port=2  VectorParamsAs1DForOutWhenUnconnected=off
  wires:
  Gain/1 -> Tem/1
  isq/1 -> Divide/1, Gain/1
  Gain1/1 -> Ter/1
  Divide/1 -> Gain1/1
  isd/1 -> Divide/2
